simulink model "ActMod_TrqCalc"  (R2016b)
settings: configuration reference "CodeGenConfigSet" (kept outside this file)
PostLoadFcn:
  | , if any(exist('dsrtsu_mdlpostloadfcn', 'file') == [2, 3, 6]), try dsrtsu_mdlpostloadfcn('Execute', bdroot); catch fprintf('Error in PostLoadFcn (dsrtsu_mdlpostloadfcn) for model "%s":\n %s\n', bdroot, lasterr); end, end,
values from neighbouring files (symbols this model uses):
  PRC_100 = fi(100,Prc_100_rate)    [init_ActMod_TrqCalc.m]    (also in init_ActMod_TrqCalc_SIL.m)
undefined symbols (not defined in the file or in its folder): EngState_conv
libraries: CXLib x1
settings Model: DSRTSU_INTERNAL_RTI_VER=480  DSRTSU_INTERNAL_RTI_TYPE=rti1104  Creator=Administrator  LastModifiedBy=zhoutinglin
settings ConfigSetRef: SourceLocation=Base Workspace

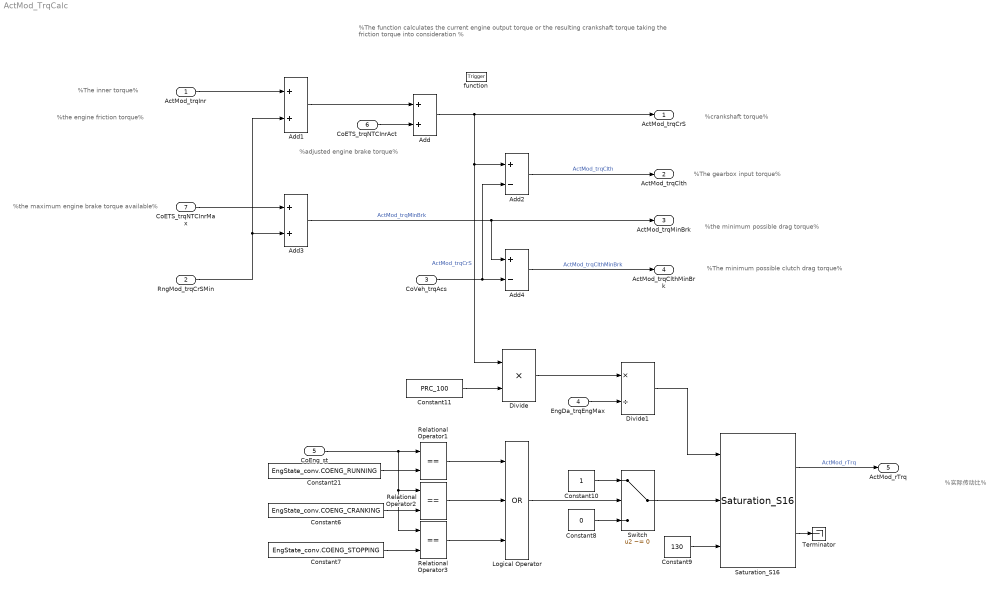
== system ActMod_TrqCalc ==
  note: %实际传动比%
  note: %The minimum possible clutch drag torque%
  note: %crankshaft torque%
  note: %the maximum engine brake torque available%
  note: %the minimum possible drag torque%
  note: %The gearbox input torque%
  note: %adjusted engine brake torque%
  note: %the engine friction torque%
  note: %The inner torque%
  note: %The function calculates the current engine output torque or
      | the resulting crankshaft torque taking the friction torque into consideration %
  ActMod_trqInr : Inport  Tag=Nm  Description=Current, back-calculated inner engine torque  OutMin=-3276.8  OutMax=3276.7  OutDataTypeStr=Trq_Nm
  RngMod_trqCrSMin : Inport  Tag=Nm  Description=minimal crankshaft torque  Port=2  OutMin=-3276.8  OutMax=3276.7  OutDataTypeStr=Trq_Nm
  CoVeh_trqAcs : Inport  Tag=Nm  Description=message for demand of accessories  Port=3  OutMin=-3276.8  OutMax=3276.7  OutDataTypeStr=Trq_Nm
  EngDa_trqEngMax : Inport  Tag=Nm  Description=Maximum engine output torque  Port=4  OutMin=-3276.8  OutMax=3276.7  OutDataTypeStr=Trq_Nm
  CoEng_st : Inport  Description=Engine coordinator state  Port=5  OutDataTypeStr=Enum: EngState_conv
  CoETS_trqNTCInrAct : Inport  Tag=Nm  Description=Actual braking torque  Port=6  OutMin=-3276.8  OutMax=3276.7  OutDataTypeStr=Trq_Nm
  CoETS_trqNTCInrMax : Inport  Tag=Nm  Description=Maximum available braking torque  Port=7  OutMin=-3276.8  OutMax=3276.7  OutDataTypeStr=Trq_Nm
  function : TriggerPort  TriggerType=function-call  VariantControl=Variant
  Add : Sum  SaturateOnIntegerOverflow=on  InputSameDT=on
  Add1 : Sum  OutDataTypeStr=Inherit: Inherit via back propagation  SaturateOnIntegerOverflow=on  InputSameDT=on
  Add2 : Sum  Inputs=+-  OutDataTypeStr=Inherit: Inherit via back propagation  SaturateOnIntegerOverflow=on  InputSameDT=on
  Add3 : Sum  OutDataTypeStr=Inherit: Inherit via back propagation  SaturateOnIntegerOverflow=on  InputSameDT=on
  Add4 : Sum  Inputs=+-  OutDataTypeStr=Inherit: Inherit via back propagation  SaturateOnIntegerOverflow=on  InputSameDT=on
  Constant10 : Constant  OutDataTypeStr=Inherit: Inherit via back propagation
  Constant11 : Constant  Value=PRC_100
  Constant21 : Constant  Value=EngState_conv.COENG_RUNNING  OutDataTypeStr=Inherit: Inherit via back propagation
  Constant6 : Constant  Value=EngState_conv.COENG_CRANKING  OutDataTypeStr=Inherit: Inherit via back propagation
  Constant7 : Constant  Value=EngState_conv.COENG_STOPPING  OutDataTypeStr=Inherit: Inherit via back propagation
  Constant8 : Constant  Value=0  OutDataTypeStr=Inherit: Inherit via back propagation
  Constant9 : Constant  Value=130  OutDataTypeStr=Inherit: Inherit via back propagation
  Divide : Product  Inputs=**  OutDataTypeStr=fixdt(1,32,8)  SaturateOnIntegerOverflow=on
  Divide1 : Product  Inputs=*/  OutDataTypeStr=Inherit: Inherit via back propagation  SaturateOnIntegerOverflow=on
  Logical Operator : Logic  Operator=OR  Inputs=3  OutDataTypeStr=boolean
  Relational Operator1 : RelationalOperator  Operator===  OutDataTypeStr=boolean  RndMeth=Simplest  InputSameDT=on
  Relational Operator2 : RelationalOperator  Operator===  OutDataTypeStr=boolean  RndMeth=Simplest  InputSameDT=on
  Relational Operator3 : RelationalOperator  Operator===  OutDataTypeStr=boolean  RndMeth=Simplest  InputSameDT=on
  Saturation_S16 : CXLib/Saturation_S16
  Switch : Switch  Criteria=u2 ~= 0  SaturateOnIntegerOverflow=on  InputSameDT=on
  Terminator : Terminator
  ActMod_trqCrS : Outport  Tag=Nm  Description=Current crankshaft torque  OutMin=-3276.8  OutMax=3276.7  OutDataTypeStr=Trq_Nm
  ActMod_trqClth : Outport  Tag=Nm  Description=actual engine torque - clutch torque  Port=2  OutMin=-3276.8  OutMax=3276.7  OutDataTypeStr=Trq_Nm
  ActMod_trqMinBrk : Outport  Tag=Nm  Description=minimum possible drag torque  Port=3  OutMin=-3276.8  OutMax=3276.7  OutDataTypeStr=Trq_Nm
  ActMod_trqClthMinBrk : Outport  Tag=Nm  Description=minimum possible clutch drag torque.  Port=4  OutMin=-3276.8  OutMax=3276.7  OutDataTypeStr=Trq_Nm
  ActMod_rTrq : Outport  Tag=%  Description=Actual engine output torque ratio  Port=5  OutMin=-300  OutMax=300  OutDataTypeStr=Prc_100_rate
  wires:
  Constant6/1 -> Relational Operator2/2
  Logical Operator/1 -> Switch/2
  Relational Operator1/1 -> Logical Operator/1
  Saturation_S16/1 -> ActMod_rTrq/1  "ActMod_rTrq"
  Saturation_S16/2 -> Terminator/1
  CoEng_st/1 -> Relational Operator1/1, Relational Operator3/1, Relational Operator2/1
  Add4/1 -> ActMod_trqClthMinBrk/1  "ActMod_trqClthMinBrk"
  Add1/1 -> Add/1
  Divide/1 -> Divide1/1
  Constant9/1 -> Saturation_S16/3
  Switch/1 -> Saturation_S16/2
  Constant8/1 -> Switch/3
  Relational Operator2/1 -> Logical Operator/2
  Constant21/1 -> Relational Operator1/2
  Constant7/1 -> Relational Operator3/2
  ActMod_trqInr/1 -> Add1/1
  Relational Operator3/1 -> Logical Operator/3
  Add2/1 -> ActMod_trqClth/1  "ActMod_trqClth"
  Constant10/1 -> Switch/1
  Add/1 -> Divide/1, Add2/1, ActMod_trqCrS/1  "ActMod_trqCrS"
  CoVeh_trqAcs/1 -> Add2/2, Add4/2
  Add3/1 -> ActMod_trqMinBrk/1, Add4/1  "ActMod_trqMinBrk"
  RngMod_trqCrSMin/1 -> Add1/2, Add3/2
  Constant11/1 -> Divide/2
  Divide1/1 -> Saturation_S16/1
  EngDa_trqEngMax/1 -> Divide1/2
  CoETS_trqNTCInrAct/1 -> Add/2
  CoETS_trqNTCInrMax/1 -> Add3/1
